simulink model "CAN_2_Legs_whileloop_johnmessingabout"  (R2021a)
settings: Solver=FixedStepAuto  StartTime=0.0  StopTime=200  FixedStep=.1  RelTol=1e-3
libraries: speedgoatlib_IO691 x5, canmsglib x4, slrealtimeutilitieslib x2
settings Model: SimulationMode=external  Creator=celwe  LastModifiedBy=johna
settings SolverCC: ConcurrentTasks=on  PositivePriorityOrder=on
settings OptimizationCC: BlockReduction=off  OptimizeBlockIOStorage=off
settings DebuggingCC: TasksWithSamePriorityMsg=none
settings HardwareCC: ProdBitPerLong=64  ProdLongLongMode=on  ProdHWDeviceType=Intel->x86-64 (Linux 64)
settings RTWCC: Description=Simulink Real-Time  SystemTargetFile=slrealtime.tlc  TemplateMakefile=slrealtime_default_tmf  Toolchain=Simulink Real-Time Toolchain  BuildConfiguration=Faster Runs  CodeExecutionProfiling=on  TargetLang=C++

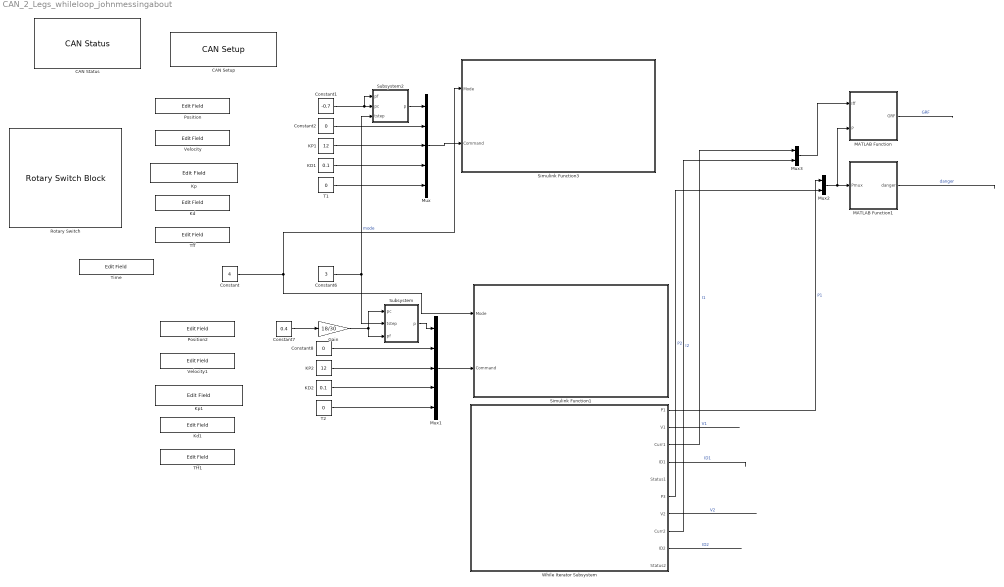
== system CAN_2_Legs_whileloop_johnmessingabout ==
  "CAN Setup " : speedgoatlib_IO691/CAN Setup   moduletype=IO691  id=1  pciSlot=-1  chn1=CAN (HS)  chn2=CAN (HS)  chn3=Disabled  chn4=Disabled  initStruct=[]  termStruct=[]  ArbitrationbdrChn1=1.0 MBaud  ArbitrationManbdrChn1=[2,8,31,8]  FdbdrChn1=5.0 MBaud  FdManbdrChn1=[2,2,5,2]  ArbitrationbdrChn2=1.0 MBaud  ArbitrationManbdrChn2=[2,8,31,8]  FdbdrChn2=5.0 MBaud  FdManbdrChn2=[2,2,5,2]  ArbitrationbdrChn3=1.0 MBaud  ArbitrationManbdrChn3=[2,8,31,8]  FdbdrChn3=5.0 MBaud  FdManbdrChn3=[2,2,5,2]  ArbitrationbdrChn4=1.0 MBaud  ArbitrationManbdrChn4=[2,8,31,8]  FdbdrChn4=5.0 MBaud  FdManbdrChn4=[2,2,5,2]  moduleInitValues=[691 1 -1 -1]
      settings: SourceProductName=Simulink Real-Time: Speedgoat I/O Blockset
  CAN Status : speedgoatlib_IO691/CAN Status  moduleId=1  sampleTime=-1  channel=1  busRecovery=Off  arrayOutput=off  controllerCpuLoad=off  controllerLiveCount=off  initModeAct=off  avgBusLoad=off  receiving=off  RxQueueEmpty=off  dataOverrunRcv=off  rxBufferLevel=off  txPending=off  dataOverrunTx=off  txBufferLevel=off  errWarnLimit=off  errPassLimit=off  errBusOff=off  busRecoveryCounter=off  busCouplingErr=off  transceiverErr=off  opMode=off  brp=off  timeSegment1=off  timeSegment2=off  synchronisationJumpWidth=off  dataTSEG1=off  dataTSEG2=off  dataSJW=off  moduleType=691  qtyStatBlk=1  ptIdx=0  isFDMod=0
      settings: SourceProductName=Simulink Real-Time: Speedgoat I/O Blockset
  Constant : Constant  Value=4
  Constant1 : Constant  Value=-0.7
  Constant2 : Constant  Value=0
  Constant6 : Constant  Value=3
  Constant7 : Constant  Value=0.4
  Constant8 : Constant  Value=0
  Gain : Gain  Gain=18/30
  KD1 : Constant  Value=0.1
  KD2 : Constant  Value=0.1
  KP1 : Constant  Value=12
  KP2 : Constant  Value=12
  Kd : EditField  LabelPosition=Hide  ShowInitialText=on  Alignment=Center
  Kd1 : EditField  LabelPosition=Hide  ShowInitialText=on  Alignment=Center
  Kp : EditField  LabelPosition=Hide  ShowInitialText=on  Alignment=Center
  Kp1 : EditField  LabelPosition=Hide  ShowInitialText=on  Alignment=Center
  MATLAB Function : MATLAB Function  TreatAsAtomicUnit=on
  MATLAB Function1 : MATLAB Function  TreatAsAtomicUnit=on
  Mux : Mux  Inputs=5
  Mux1 : Mux  Inputs=5
  Mux2 : Mux  Inputs=2
  Mux3 : Mux  Inputs=2
  Position : EditField  LabelPosition=Hide  ShowInitialText=on  Alignment=Center
  Position2 : EditField  LabelPosition=Hide  ShowInitialText=on  Alignment=Center
  Rotary Switch : RotarySwitchBlock
      settings: Values={{'Zero', 'Init', 'Command', 'Deinit'}, [1 2 3 4]}
  Simulink Function1 : Subsystem  TreatAsAtomicUnit=on
  Simulink Function3 : Subsystem  TreatAsAtomicUnit=on
  Subsystem : Subsystem
  Subsystem2 : Subsystem
  T1 : Constant  Value=0
  T2 : Constant  Value=0
  Tff : EditField  LabelPosition=Hide  ShowInitialText=on  Alignment=Center
  Tff1 : EditField  LabelPosition=Hide  ShowInitialText=on  Alignment=Center
  Time : EditField  LabelPosition=Hide  ShowInitialText=on  Alignment=Center
  Velocity : EditField  LabelPosition=Hide  ShowInitialText=on  Alignment=Center
  Velocity1 : EditField  LabelPosition=Hide  ShowInitialText=on  Alignment=Center
  While Iterator Subsystem : Subsystem  TreatAsAtomicUnit=on
  wires:
  Mux/1 -> Simulink Function3/2(Command)
  Constant2/1 -> Mux/2
  Constant1/1 -> Subsystem2/1(pf), Subsystem2/2(pc)
  KP1/1 -> Mux/3
  KD1/1 -> Mux/4
  T1/1 -> Mux/5
  KD2/1 -> Mux1/4
  Constant8/1 -> Mux1/2
  Mux1/1 -> Simulink Function1/2(Command)
  KP2/1 -> Mux1/3
  Constant/1 -> Simulink Function3/1(Mode), Simulink Function1/1(Mode)  "mode"
  T2/1 -> Mux1/5
  Mux2/1 -> MATLAB Function/2(P), MATLAB Function1/1(Pmux)
  MATLAB Function/1(GRF) -> ?  "GRF"
  MATLAB Function1/1(danger) -> ?  "danger"
  Subsystem2/1(p) -> Mux/1
  Subsystem/1(p) -> Mux1/1
  Constant6/1 -> Subsystem/2(tstep), Subsystem2/3(tstep)
  Gain/1 -> Subsystem/1(pc), Subsystem/3(pf)
  Constant7/1 -> Gain/1
  While Iterator Subsystem/1(P1) -> Mux2/1  "P1"
  While Iterator Subsystem/2(V1) -> ?  "V1"
  While Iterator Subsystem/3(Curr1) -> Mux3/1  "I1"
  While Iterator Subsystem/4(ID1) -> ?  "ID1"
  While Iterator Subsystem/6(P3) -> Mux2/2  "P2"
  While Iterator Subsystem/7(V2) -> ?  "V2"
  While Iterator Subsystem/8(Curr2) -> Mux3/2  "I2"
  While Iterator Subsystem/9(ID2) -> ?  "ID2"
  Mux3/1 -> MATLAB Function/1(Iff)

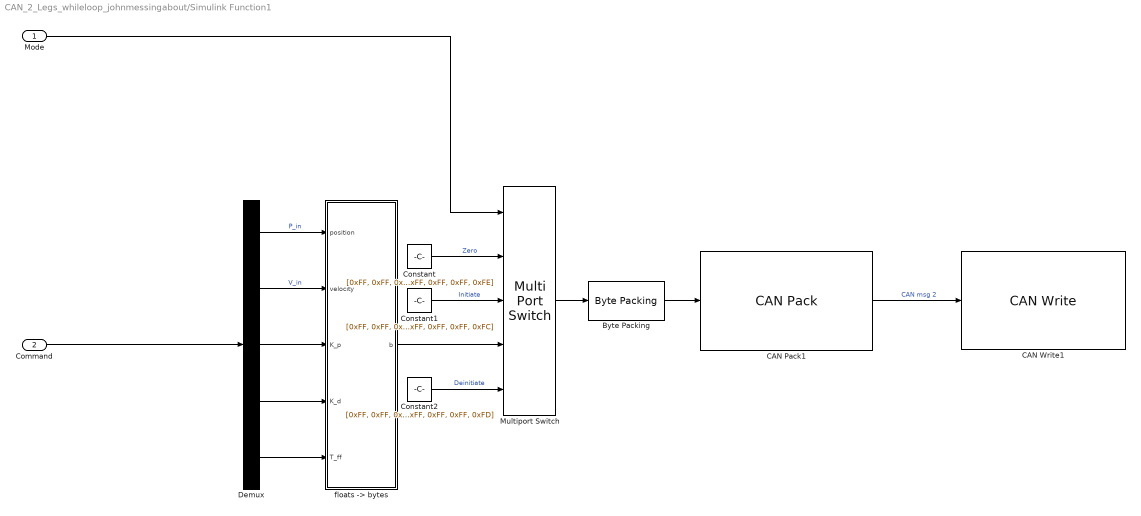
== system CAN_2_Legs_whileloop_johnmessingabout/Simulink Function1 ==
  Mode : Inport
  Command : Inport  Port=2
  Byte Packing : slrealtimeutilitieslib/Byte Packing  MaskPackedDataType=uint8  MaskUnpackedDataTypes={['uint8']}  MaskAlignment=1
  CAN Pack1 : canmsglib/CAN Pack  MsgList=(none)  MsgName=CAN Msg  MsgIDType=Standard (11-bit identifier)  MsgIdentifier=2  MsgLength=8  Remote=off  ApplyMinMax=off  BusOutput=off  SignalInfo={ 'b1', '0', '8', 'LE', 'unsigned', 'Standard', '0', '1', '0', '-Inf', 'Inf'; 'b2', '8', '8', 'LE', 'unsigned', 'Standard', '0', '1', '0', '-Inf', 'Inf'; 'b3', '16', '8', 'LE', 'unsigned', 'Standard', '0', '1', '0', '-Inf', 'Inf'; 'b4', '24', '8', 'LE', 'unsigned', 'Standard', '0', '1', '0', '-Inf', 'Inf'; 'b5', '32', '8', 'LE', 'unsigned', 'Standard', '0', '1', '0', '-Inf', 'Inf'; 'b6', '40', '8', 'LE', 'unsigned', 'Standard', '0', '1', '0', '-Inf', 'Inf'; 'b7', '48', '8', 'LE', 'unsigned', 'Standard', '0', '1', '0', '-Inf', 'Inf'; 'b8', '56', '8', 'LE', 'unsigned', 'Standard', '0', '1', '0', '-Inf', 'Inf' }
      settings: SourceProductBaseCode=ME,XP,VN  DataFormat=raw data
  CAN Write1 : speedgoatlib_IO691/CAN Write  id=1  ts=-1  channel=1  messageType=CAN  enableStatusPort=off  canType=CAN (HS)  initValues=[691 1 -1 0 1 1 0]
      settings: SourceProductName=Simulink Real-Time: Speedgoat I/O Blockset
  Constant : Constant  Value=[0xFF, 0xFF, 0xFF, 0xFF, 0xFF, 0xFF, 0xFF, 0xFE]
  Constant1 : Constant  Value=[0xFF, 0xFF, 0xFF, 0xFF, 0xFF, 0xFF, 0xFF, 0xFC]
  Constant2 : Constant  Value=[0xFF, 0xFF, 0xFF, 0xFF, 0xFF, 0xFF, 0xFF, 0xFD]
  Demux : Demux  Outputs=5
  Multiport Switch : MultiPortSwitch  Inputs=4
  "floats -> bytes" : MATLAB Function  TreatAsAtomicUnit=on
  wires:
  Demux/5 -> "floats -> bytes"/5(T_ff)
  Multiport Switch/1 -> Byte Packing/1
  Demux/4 -> "floats -> bytes"/4(K_d)
  Demux/1 -> "floats -> bytes"/1(position)  "P_in"
  Constant/1 -> Multiport Switch/2  "Zero"
  Demux/2 -> "floats -> bytes"/2(velocity)  "V_in"
  Constant2/1 -> Multiport Switch/5  "Deinitiate"
  CAN Pack1/1 -> CAN Write1/1  "CAN msg 2"
  Byte Packing/1 -> CAN Pack1/1
  Constant1/1 -> Multiport Switch/3  "Initiate"
  "floats -> bytes"/1(b) -> Multiport Switch/4
  Demux/3 -> "floats -> bytes"/3(K_p)
  Mode/1 -> Multiport Switch/1
  Command/1 -> Demux/1

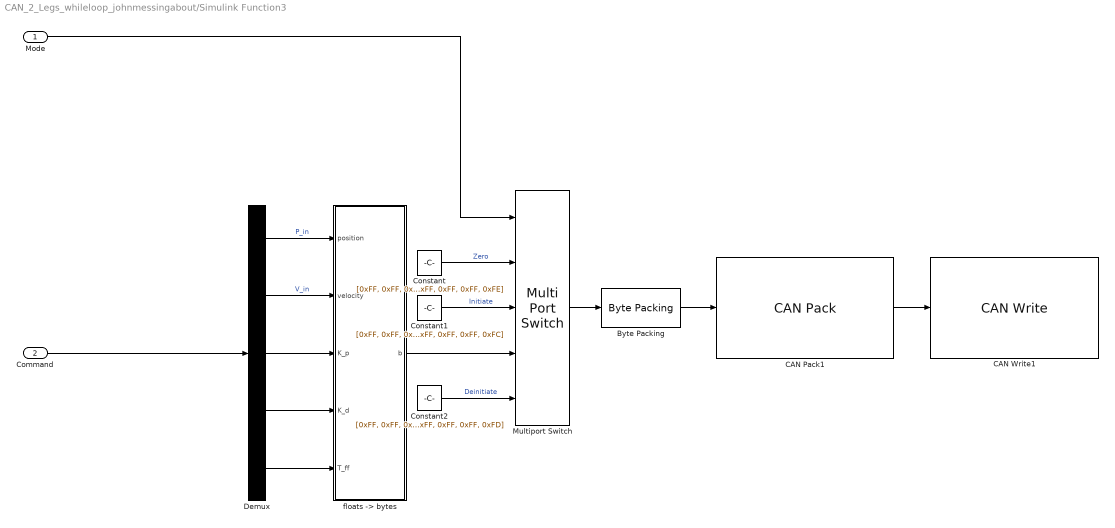
== system CAN_2_Legs_whileloop_johnmessingabout/Simulink Function3 ==
  Mode : Inport
  Command : Inport  Port=2
  Byte Packing : slrealtimeutilitieslib/Byte Packing  MaskPackedDataType=uint8  MaskUnpackedDataTypes={['uint8']}  MaskAlignment=1
  CAN Pack1 : canmsglib/CAN Pack  MsgList=(none)  MsgName=CAN Msg  MsgIDType=Standard (11-bit identifier)  MsgIdentifier=1  MsgLength=8  Remote=off  ApplyMinMax=off  BusOutput=off  SignalInfo={ 'b1', '0', '8', 'LE', 'unsigned', 'Standard', '0', '1', '0', '-Inf', 'Inf'; 'b2', '8', '8', 'LE', 'unsigned', 'Standard', '0', '1', '0', '-Inf', 'Inf'; 'b3', '16', '8', 'LE', 'unsigned', 'Standard', '0', '1', '0', '-Inf', 'Inf'; 'b4', '24', '8', 'LE', 'unsigned', 'Standard', '0', '1', '0', '-Inf', 'Inf'; 'b5', '32', '8', 'LE', 'unsigned', 'Standard', '0', '1', '0', '-Inf', 'Inf'; 'b6', '40', '8', 'LE', 'unsigned', 'Standard', '0', '1', '0', '-Inf', 'Inf'; 'b7', '48', '8', 'LE', 'unsigned', 'Standard', '0', '1', '0', '-Inf', 'Inf'; 'b8', '56', '8', 'LE', 'unsigned', 'Standard', '0', '1', '0', '-Inf', 'Inf' }
      settings: SourceProductBaseCode=ME,XP,VN  DataFormat=raw data
  CAN Write1 : speedgoatlib_IO691/CAN Write  id=1  ts=-1  channel=1  messageType=CAN  enableStatusPort=off  canType=CAN (HS)  initValues=[691 1 -1 0 1 1 0]
      settings: SourceProductName=Simulink Real-Time: Speedgoat I/O Blockset
  Constant : Constant  Value=[0xFF, 0xFF, 0xFF, 0xFF, 0xFF, 0xFF, 0xFF, 0xFE]
  Constant1 : Constant  Value=[0xFF, 0xFF, 0xFF, 0xFF, 0xFF, 0xFF, 0xFF, 0xFC]
  Constant2 : Constant  Value=[0xFF, 0xFF, 0xFF, 0xFF, 0xFF, 0xFF, 0xFF, 0xFD]
  Demux : Demux  Outputs=5
  Multiport Switch : MultiPortSwitch  Inputs=4
  "floats -> bytes" : MATLAB Function  TreatAsAtomicUnit=on
  wires:
  Demux/5 -> "floats -> bytes"/5(T_ff)
  Multiport Switch/1 -> Byte Packing/1
  Demux/4 -> "floats -> bytes"/4(K_d)
  Demux/1 -> "floats -> bytes"/1(position)  "P_in"
  Constant/1 -> Multiport Switch/2  "Zero"
  Demux/2 -> "floats -> bytes"/2(velocity)  "V_in"
  Constant2/1 -> Multiport Switch/5  "Deinitiate"
  CAN Pack1/1 -> CAN Write1/1
  Byte Packing/1 -> CAN Pack1/1
  Constant1/1 -> Multiport Switch/3  "Initiate"
  "floats -> bytes"/1(b) -> Multiport Switch/4
  Demux/3 -> "floats -> bytes"/3(K_p)
  Mode/1 -> Multiport Switch/1
  Command/1 -> Demux/1

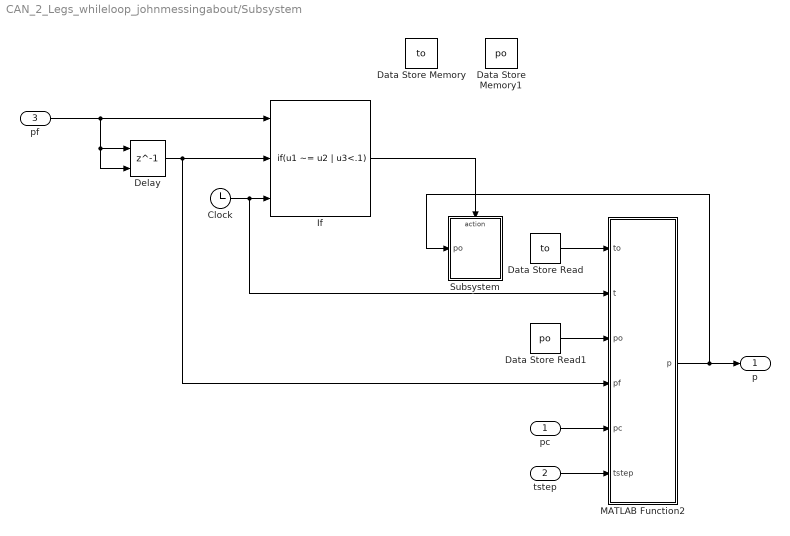
== system CAN_2_Legs_whileloop_johnmessingabout/Subsystem ==
  pc : Inport
  tstep : Inport  Port=2
  pf : Inport  Port=3
  Clock : Clock
  Data Store Memory : DataStoreMemory  DataStoreName=to  ReadBeforeWriteMsg=warning  WriteAfterWriteMsg=warning  WriteAfterReadMsg=warning  ShowAdditionalParam=off
  Data Store Memory1 : DataStoreMemory  DataStoreName=po  ReadBeforeWriteMsg=warning  WriteAfterWriteMsg=warning  WriteAfterReadMsg=warning  ShowAdditionalParam=off
  Data Store Read : DataStoreRead  DataStoreName=to  IndexOptions=Index vector (dialog)  Indices=1  OutputSizes=1
  Data Store Read1 : DataStoreRead  DataStoreName=po  IndexOptions=Index vector (dialog)  Indices=1  OutputSizes=1
  Delay : Delay  DelayLength=1  InitialConditionSource=Input port
      settings: InputPortMap=u0,p4
  If : If  NumInputs=3  IfExpression=u1 ~= u2 | u3<.1  ShowElse=off
  MATLAB Function2 : MATLAB Function  TreatAsAtomicUnit=on
  Subsystem : Subsystem
  p : Outport
  wires:
  Clock/1 -> MATLAB Function2/2(t), If/3
  MATLAB Function2/1(p) -> Subsystem/1(po), p/1
  tstep/1 -> MATLAB Function2/6(tstep)
  pf/1 -> Delay/2, Delay/1, If/1
  If/1 -> Subsystem/Action
  Delay/1 -> MATLAB Function2/4(pf), If/2
  Data Store Read/1 -> MATLAB Function2/1(to)
  Data Store Read1/1 -> MATLAB Function2/3(po)
  pc/1 -> MATLAB Function2/5(pc)

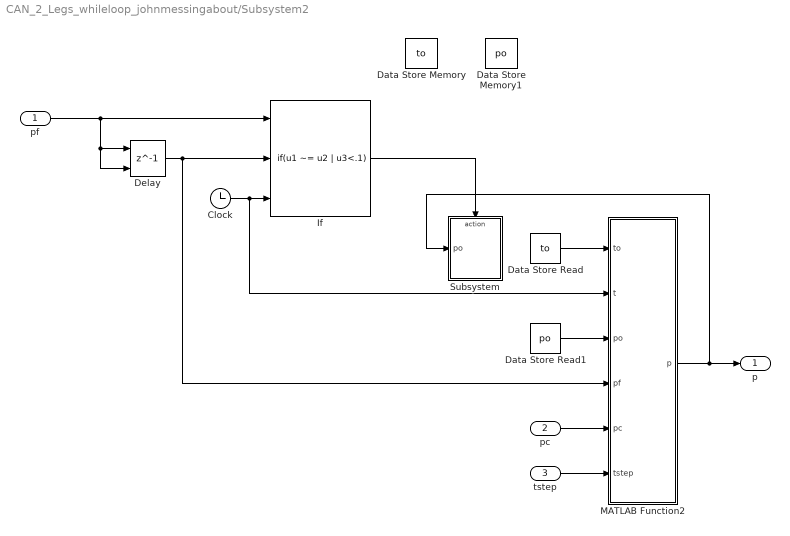
== system CAN_2_Legs_whileloop_johnmessingabout/Subsystem2 ==
  pf : Inport
  pc : Inport  Port=2
  tstep : Inport  Port=3
  Clock : Clock
  Data Store Memory : DataStoreMemory  DataStoreName=to  ReadBeforeWriteMsg=warning  WriteAfterWriteMsg=warning  WriteAfterReadMsg=warning  ShowAdditionalParam=off
  Data Store Memory1 : DataStoreMemory  DataStoreName=po  ReadBeforeWriteMsg=warning  WriteAfterWriteMsg=warning  WriteAfterReadMsg=warning  ShowAdditionalParam=off
  Data Store Read : DataStoreRead  DataStoreName=to  IndexOptions=Index vector (dialog)  Indices=1  OutputSizes=1
  Data Store Read1 : DataStoreRead  DataStoreName=po  IndexOptions=Index vector (dialog)  Indices=1  OutputSizes=1
  Delay : Delay  DelayLength=1  InitialConditionSource=Input port
      settings: InputPortMap=u0,p4
  If : If  NumInputs=3  IfExpression=u1 ~= u2 | u3<.1  ShowElse=off
  MATLAB Function2 : MATLAB Function  TreatAsAtomicUnit=on
  Subsystem : Subsystem
  p : Outport
  wires:
  Clock/1 -> MATLAB Function2/2(t), If/3
  MATLAB Function2/1(p) -> Subsystem/1(po), p/1
  tstep/1 -> MATLAB Function2/6(tstep)
  pf/1 -> Delay/2, Delay/1, If/1
  If/1 -> Subsystem/Action
  Delay/1 -> MATLAB Function2/4(pf), If/2
  Data Store Read/1 -> MATLAB Function2/1(to)
  Data Store Read1/1 -> MATLAB Function2/3(po)
  pc/1 -> MATLAB Function2/5(pc)

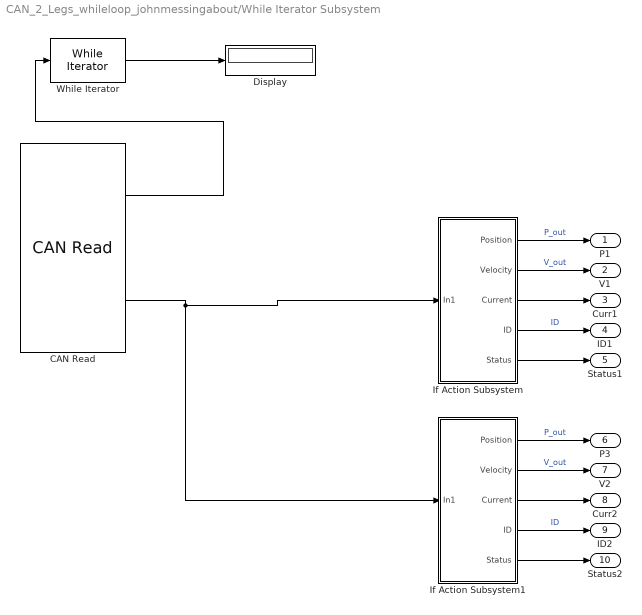
== system CAN_2_Legs_whileloop_johnmessingabout/While Iterator Subsystem ==
  CAN Read : speedgoatlib_IO691/CAN Read  id=1  ts=-1  channel=1  messageType=CAN  canType=CAN (HS)  initValues=[691 1 -1 0 1 1]
      settings: SourceProductName=Simulink Real-Time: Speedgoat I/O Blockset
  Display : Display
  If Action Subsystem : Subsystem  TreatAsAtomicUnit=on
  If Action Subsystem1 : Subsystem  TreatAsAtomicUnit=on
  While Iterator : WhileIterator  MaxIters=-1  WhileBlockType=do-while  ResetStates=reset  ShowIterationPort=on
  P1 : Outport
  V1 : Outport  Port=2
  Curr1 : Outport  Port=3
  ID1 : Outport  Port=4
  Status1 : Outport  Port=5
  P3 : Outport  Port=6
  V2 : Outport  Port=7
  Curr2 : Outport  Port=8
  ID2 : Outport  Port=9
  Status2 : Outport  Port=10
  wires:
  CAN Read/1 -> While Iterator/1
  CAN Read/2 -> If Action Subsystem1/1(In1), If Action Subsystem/1(In1)
  If Action Subsystem/1(Position) -> P1/1  "P_out"
  If Action Subsystem/2(Velocity) -> V1/1  "V_out"
  If Action Subsystem/3(Current) -> Curr1/1
  If Action Subsystem/4(ID) -> ID1/1  "ID"
  If Action Subsystem/5(Status) -> Status1/1
  If Action Subsystem1/5(Status) -> Status2/1
  If Action Subsystem1/4(ID) -> ID2/1  "ID"
  If Action Subsystem1/1(Position) -> P3/1  "P_out"
  If Action Subsystem1/3(Current) -> Curr2/1
  If Action Subsystem1/2(Velocity) -> V2/1  "V_out"
  While Iterator/1 -> Display/1

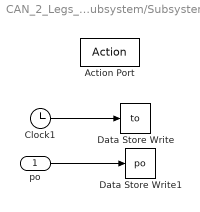
== system CAN_2_Legs_whileloop_johnmessingabout/Subsystem/Subsystem ==
  po : Inport
  Action Port : ActionPort  ActionPortLabel=if(u1 ~= u2 | u3<.1)
  Clock1 : Clock
  Data Store Write : DataStoreWrite  DataStoreName=to  IndexOptions=Index vector (dialog)  Indices=1  OutputSizes=1
  Data Store Write1 : DataStoreWrite  DataStoreName=po  IndexOptions=Index vector (dialog)  Indices=1  OutputSizes=1
  wires:
  Clock1/1 -> Data Store Write/1
  po/1 -> Data Store Write1/1

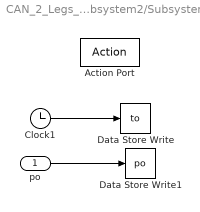
== system CAN_2_Legs_whileloop_johnmessingabout/Subsystem2/Subsystem ==
  po : Inport
  Action Port : ActionPort  ActionPortLabel=if(u1 ~= u2 | u3<.1)
  Clock1 : Clock
  Data Store Write : DataStoreWrite  DataStoreName=to  IndexOptions=Index vector (dialog)  Indices=1  OutputSizes=1
  Data Store Write1 : DataStoreWrite  DataStoreName=po  IndexOptions=Index vector (dialog)  Indices=1  OutputSizes=1
  wires:
  Clock1/1 -> Data Store Write/1
  po/1 -> Data Store Write1/1

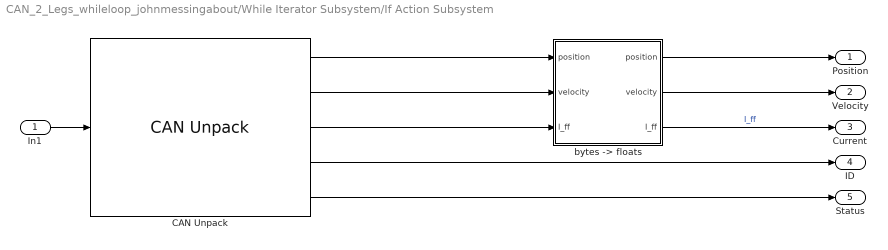
== system CAN_2_Legs_whileloop_johnmessingabout/While Iterator Subsystem/If Action Subsystem ==
  In1 : Inport
  CAN Unpack : canmsglib/CAN Unpack  MsgList=(none)  MsgName=CAN Msg  MsgIDType=Standard (11-bit identifier)  MsgIdentifier=1  MsgLength=6  SignalInfo={ 'position', '16', '16', 'BE', 'unsigned', 'Standard', '0', '1', '0', '0', '65535'; 'velocity', '36', '12', 'BE', 'unsigned', 'Standard', '0', '1', '0', '0', '4095'; 'current', '40', '12', 'BE', 'unsigned', 'Standard', '0', '1', '0', '0', '4095'; 'id', '0', '8', 'BE', 'unsigned', 'Standard', '0', '1', '0', '0', '255' }  IDPort=off  TimestampPort=off  ErrorPort=off  RemotePort=off  LengthPort=off  StatusPort=on  ApplyMinMax=off
      settings: SourceProductBaseCode=ME,XP,VN
  "bytes -> floats" : MATLAB Function  TreatAsAtomicUnit=on
  Position : Outport
  Velocity : Outport  Port=2
  Current : Outport  Port=3
  ID : Outport  Port=4
  Status : Outport  Port=5
  wires:
  CAN Unpack/5 -> Status/1
  CAN Unpack/3 -> "bytes -> floats"/3("I_ff ")
  CAN Unpack/4 -> ID/1
  "bytes -> floats"/2(velocity) -> Velocity/1
  "bytes -> floats"/3(I_ff) -> Current/1  "I_ff"
  CAN Unpack/2 -> "bytes -> floats"/2("velocity ")
  In1/1 -> CAN Unpack/1
  CAN Unpack/1 -> "bytes -> floats"/1("position ")
  "bytes -> floats"/1(position) -> Position/1

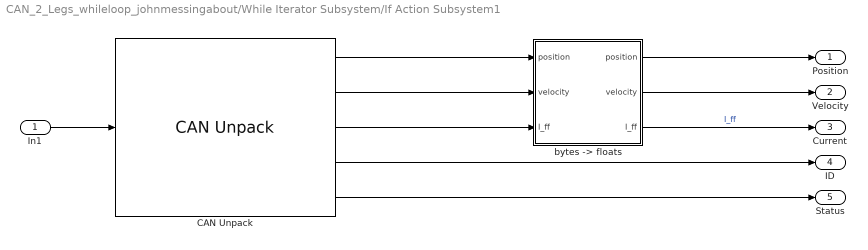
== system CAN_2_Legs_whileloop_johnmessingabout/While Iterator Subsystem/If Action Subsystem1 ==
  In1 : Inport
  CAN Unpack : canmsglib/CAN Unpack  MsgList=(none)  MsgName=CAN Msg  MsgIDType=Standard (11-bit identifier)  MsgIdentifier=2  MsgLength=6  SignalInfo={ 'position', '16', '16', 'BE', 'unsigned', 'Standard', '0', '1', '0', '0', '65535'; 'velocity', '36', '12', 'BE', 'unsigned', 'Standard', '0', '1', '0', '0', '4095'; 'current', '40', '12', 'BE', 'unsigned', 'Standard', '0', '1', '0', '0', '4095'; 'id', '0', '8', 'BE', 'unsigned', 'Standard', '0', '1', '0', '0', '255' }  IDPort=off  TimestampPort=off  ErrorPort=off  RemotePort=off  LengthPort=off  StatusPort=on  ApplyMinMax=off
      settings: SourceProductBaseCode=ME,XP,VN
  "bytes -> floats" : MATLAB Function  TreatAsAtomicUnit=on
  Position : Outport
  Velocity : Outport  Port=2
  Current : Outport  Port=3
  ID : Outport  Port=4
  Status : Outport  Port=5
  wires:
  CAN Unpack/5 -> Status/1
  CAN Unpack/1 -> "bytes -> floats"/1("position ")
  CAN Unpack/3 -> "bytes -> floats"/3("I_ff ")
  "bytes -> floats"/1(position) -> Position/1
  CAN Unpack/4 -> ID/1
  "bytes -> floats"/2(velocity) -> Velocity/1
  "bytes -> floats"/3(I_ff) -> Current/1  "I_ff"
  CAN Unpack/2 -> "bytes -> floats"/2("velocity ")
  In1/1 -> CAN Unpack/1

== matlab function CAN_2_Legs_whileloop_johnmessingabout/While Iterator Subsystem/If Action Subsystem1/bytes -> floats ==
  data: position input; position output; velocity output; I_ff output; velocity input; I_ff input
function [position, velocity, I_ff] = fcn(position, velocity, I_ff)

P_MIN  =-95.5;  % [rad]
P_MAX  = 95.5;  % [rad]
V_MIN  =-45;    % [rad/s]
V_MAX  = 45;    % [rad/s]
I_MIN  =-40;    % []
I_MAX  = 40;    % []

position = position*(P_MAX  - P_MIN)/65535+ P_MIN;
velocity = velocity*(V_MAX  - V_MIN)/4095 + V_MIN;
I_ff     = I_ff*(I_MAX  - I_MIN)/4095 + I_MIN;

== matlab function CAN_2_Legs_whileloop_johnmessingabout/While Iterator Subsystem/If Action Subsystem/bytes -> floats ==
  data: position input; position output; velocity output; I_ff output; velocity input; I_ff input
function [position, velocity, I_ff] = fcn(position, velocity, I_ff)

P_MIN  =-95.5;  % [rad]
P_MAX  = 95.5;  % [rad]
V_MIN  =-45;    % [rad/s]
V_MAX  = 45;    % [rad/s]
I_MIN  =-40;    % []
I_MAX  = 40;    % []

position = position*(P_MAX  - P_MIN)/65535+ P_MIN;
velocity = velocity*(V_MAX  - V_MIN)/4095 + V_MIN;
I_ff     = I_ff*(I_MAX  - I_MIN)/4095 + I_MIN;

== matlab function CAN_2_Legs_whileloop_johnmessingabout/Simulink Function1/floats -> bytes ==
  data: position input; b output uint8 size=8; velocity input; K_p input; K_d input; T_ff input
function b = fcn(position, velocity, K_p, K_d, T_ff)

P_MIN  =-95.5;  % [rad]
P_MAX  = 95.5;  % [rad]
V_MIN  =-45;    % [rad/s] 30 to 45
V_MAX  = 45;    % [rad/s]
KP_MIN = 0;     % [Nm/rad]
KP_MAX = 500;   % [Nm/rad]
KD_MIN = 0;     % [Nm*s/rad
KD_MAX = 5;     % [Nm*s/rad
T_MIN  =-18;    % [Nm]
T_MAX  = 18;    % [Nm]

position = floor((max(min(position,P_MAX) ,P_MIN)  - P_MIN )*65535/(P_MAX  - P_MIN));
velocity = floor((max(min(velocity,V_MAX) ,V_MIN)  - V_MIN )*4095 /(V_MAX  - V_MIN));
K_p      = floor((max(min(K_p     ,KP_MAX),KP_MIN) - KP_MIN)*4095 /(KP_MAX - KP_MIN));
K_d      = floor((max(min(K_d     ,V_MAX) ,V_MIN)  - KD_MIN)*4095 /(KD_MAX - KD_MIN));
T_ff     = floor((max(min(T_ff    ,V_MAX) ,V_MIN)  - T_MIN )*4095 /(T_MAX  - T_MIN));

p  = dec2bin(position);
p  = [repmat('0', 1, 16-length(p)),p];
v  = dec2bin(velocity);
v  = [repmat('0', 1, 12-length(v)),v];
kp = dec2bin(K_p);
kp  = [repmat('0', 1, 12-length(kp)),kp];
kd = dec2bin(K_d);
kd  = [repmat('0', 1, 12-length(kd)),kd];
t  = dec2bin(T_ff);
t  = [repmat('0', 1, 12-length(t)),t];

B = repmat('0', 8, 8);

B(1,:) = p(1:8);
B(2,:) = p(9:16);
B(3,:) = v(1:8);
B(4,:) = [v(9:12),kp(1:4)];
B(5,:) = kp(5:12);
B(6,:) = kd(1:8);
B(7,:) = [kd(9:12),t(1:4)];
B(8,:) = t(5:12);

B  = bin2dec(B);

b = uint8(B);

== matlab function CAN_2_Legs_whileloop_johnmessingabout/MATLAB Function ==
  data: Iff input; P input; GRF output
function GRF = isGRF(Iff,P)
    GRF = 0;
    threshhold1 = 2.25;
    threshhold2 = 1.8;
    
    P1 = P(1);
    P2 = P(2);
    
    Iff1 = Iff(1);
    Iff2 = Iff(2);
    
    if(((P1<0 && threshhold1<Iff1)&& (P2>0 && -threshhold2>Iff2))|| ((P1>0 && -threshhold1>Iff1) && (P2<0 && threshhold2<Iff2)))
        GRF = 1;
    end

== matlab function CAN_2_Legs_whileloop_johnmessingabout/Simulink Function3/floats -> bytes ==
  data: position input; b output uint8 size=8; velocity input; K_p input; K_d input; T_ff input
function b = fcn(position, velocity, K_p, K_d, T_ff)

P_MIN  =-95.5;  % [rad]
P_MAX  = 95.5;  % [rad]
V_MIN  =-45;    % [rad/s] 30 to 45
V_MAX  = 45;    % [rad/s]
KP_MIN = 0;     % [Nm/rad]
KP_MAX = 500;   % [Nm/rad]
KD_MIN = 0;     % [Nm*s/rad
KD_MAX = 5;     % [Nm*s/rad
T_MIN  =-18;    % [Nm]
T_MAX  = 18;    % [Nm]

position = floor((max(min(position,P_MAX) ,P_MIN)  - P_MIN )*65535/(P_MAX  - P_MIN));
velocity = floor((max(min(velocity,V_MAX) ,V_MIN)  - V_MIN )*4095 /(V_MAX  - V_MIN));
K_p      = floor((max(min(K_p     ,KP_MAX),KP_MIN) - KP_MIN)*4095 /(KP_MAX - KP_MIN));
K_d      = floor((max(min(K_d     ,V_MAX) ,V_MIN)  - KD_MIN)*4095 /(KD_MAX - KD_MIN));
T_ff     = floor((max(min(T_ff    ,V_MAX) ,V_MIN)  - T_MIN )*4095 /(T_MAX  - T_MIN));

p  = dec2bin(position);
p  = [repmat('0', 1, 16-length(p)),p];
v  = dec2bin(velocity);
v  = [repmat('0', 1, 12-length(v)),v];
kp = dec2bin(K_p);
kp  = [repmat('0', 1, 12-length(kp)),kp];
kd = dec2bin(K_d);
kd  = [repmat('0', 1, 12-length(kd)),kd];
t  = dec2bin(T_ff);
t  = [repmat('0', 1, 12-length(t)),t];

B = repmat('0', 8, 8);

B(1,:) = p(1:8);
B(2,:) = p(9:16);
B(3,:) = v(1:8);
B(4,:) = [v(9:12),kp(1:4)];
B(5,:) = kp(5:12);
B(6,:) = kd(1:8);
B(7,:) = [kd(9:12),t(1:4)];
B(8,:) = t(5:12);

B  = bin2dec(B);

b = uint8(B);

== matlab function CAN_2_Legs_whileloop_johnmessingabout/MATLAB Function1 ==
  data: Pmux input; danger output
function danger = isDanger(Pmux)
    % Pmux position matrix radians
    %       [p(ID1),p(ID2),p(ID3),p(IDN)]
    
    p1Max = .5; 
    p1Min = -.5;
    p2Max = .5;
    p2Min = -.5;
    
    P1 = Pmux(1:2:end);
    P2 = Pmux(2:2:end);
    
    
    danger = 0;
    if((0<sum(P1>=p1Max + P1<=p1Min)) || (0<sum(P2>=p2Max + P2<=p2Min)))
        danger = 1;
    end

== matlab function CAN_2_Legs_whileloop_johnmessingabout/Subsystem2/MATLAB Function2 ==
  data: to input; p output; t input; po input; pf input; pc input; tstep input
function p = ramp(to,t,po,pf,pc, tstep)
    slope = (pf - po)/tstep;
    p = po + slope*(t-to);
    if((p > pf&& slope>0) || (p < pf && slope<0))
        p = pf;
    end
    if(t==0)
        p = pc;
    end

== matlab function CAN_2_Legs_whileloop_johnmessingabout/Subsystem/MATLAB Function2 ==
  data: to input; p output; t input; po input; pf input; pc input; tstep input
function p = ramp(to,t,po,pf,pc, tstep)
    slope = (pf - po)/tstep;
    p = po + slope*(t-to);
    if((p > pf&& slope>0) || (p < pf && slope<0))
        p = pf;
    end
    if(t==0)
        p = pc;
    end
